simulink model "VehCo"  (R2020b)
settings: configuration reference "cs_ert" (kept outside this file)
settings Model: DataDictionary=VehCo.sldd  EnableAccessToBaseWorkspace=off  Creator=zhoutinglin  LastModifiedBy=zhoutinglin
settings ConfigSetRef: SourceName=cs_ert

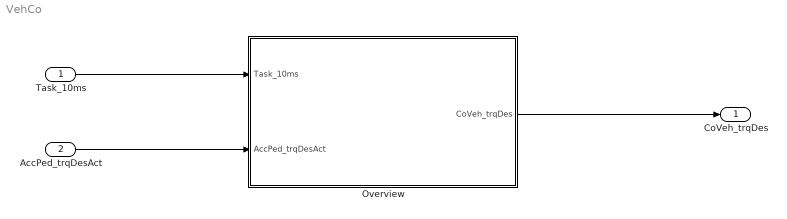
== system VehCo ==
  Task_10ms : Inport  OutputFunctionCall=on
  AccPed_trqDesAct : Inport  Port=2
  Overview : Subsystem
  CoVeh_trqDes : Outport
  wires:
  Task_10ms/1 -> Overview/1(Task_10ms)
  AccPed_trqDesAct/1 -> Overview/2(AccPed_trqDesAct)
  Overview/1(CoVeh_trqDes) -> CoVeh_trqDes/1

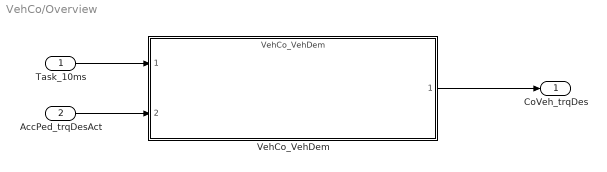
== system VehCo/Overview ==
  Task_10ms : Inport
  AccPed_trqDesAct : Inport  Port=2
  VehCo_VehDem : ModelReference  ModelNameDialog=VehCo_VehDem  SimulationMode=Normal  ScheduleRates=on  ModelReferenceVersion=1.56
  CoVeh_trqDes : Outport  VectorParamsAs1DForOutWhenUnconnected=off
  wires:
  VehCo_VehDem/1 -> CoVeh_trqDes/1
  AccPed_trqDesAct/1 -> VehCo_VehDem/2
  Task_10ms/1 -> VehCo_VehDem/1
